simulink model "BLDC_motor"  (R2020b)
settings: Solver=VariableStepAuto  StartTime=0.0  StopTime=10.0  RelTol=1e-3
values from neighbouring files (symbols this model uses):
  f1 = 1    [costant_declaration.m]
  f2 = 2    [costant_declaration.m]
  f3 = 3    [costant_declaration.m]
  J = 0.005    [costant_declaration.m]
  ke = 0.5    [costant_declaration.m]
  kf = 1.38e-8    (= 1.38e-08)    [costant_declaration.m]
  L = 0.091e-3    (= 9.1e-05)    [costant_declaration.m]
  R = 12.50    (= 12.5)    [costant_declaration.m]
undefined symbols (not defined in the file or in its folder): Te, TL
settings Model: Creator=shraddha  LastModifiedBy=shraddha

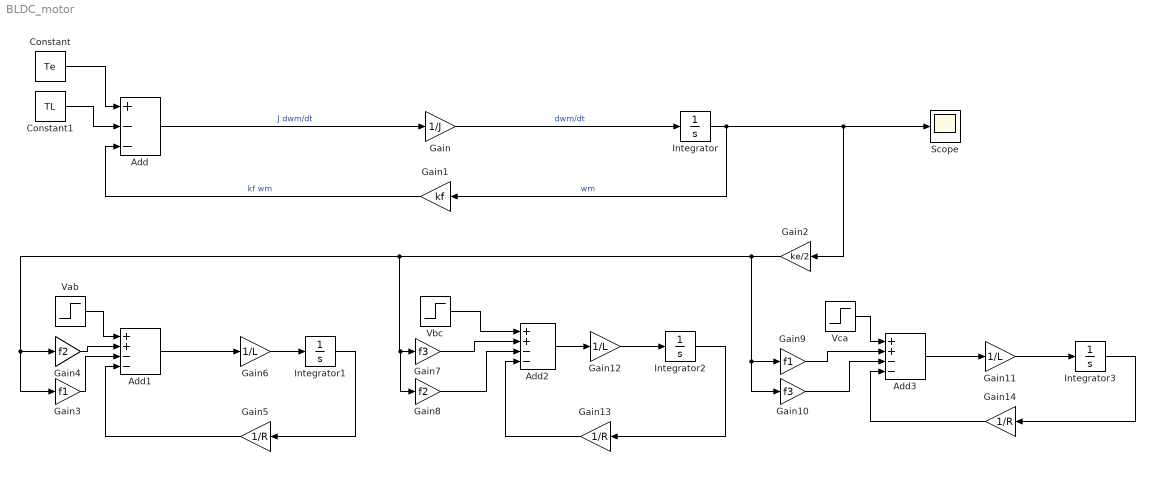
== system BLDC_motor ==
  Add : Sum  Inputs=+--
  Add1 : Sum  Inputs=++--
  Add2 : Sum  Inputs=++--
  Add3 : Sum  Inputs=++--
  Constant : Constant  Value=Te
  Constant1 : Constant  Value=TL
  Gain : Gain  Gain=1/J
  Gain1 : Gain  Gain=kf
  Gain10 : Gain  Gain=f3
  Gain11 : Gain  Gain=1/L
  Gain12 : Gain  Gain=1/L
  Gain13 : Gain  Gain=1/R
  Gain14 : Gain  Gain=1/R
  Gain2 : Gain  Gain=ke/2
  Gain3 : Gain  Gain=f1
  Gain4 : Gain  Gain=f2
  Gain5 : Gain  Gain=1/R
  Gain6 : Gain  Gain=1/L
  Gain7 : Gain  Gain=f3
  Gain8 : Gain  Gain=f2
  Gain9 : Gain  Gain=f1
  Integrator{,1..3} (4 alike) : Integrator
  Scope : Scope
  Vab : Step  SampleTime=0
  Vbc : Step  SampleTime=0
  Vca : Step  SampleTime=0
  wires:
  Add/1 -> Gain/1  "J dwm/dt"
  Gain/1 -> Integrator/1  "dwm/dt"
  Integrator/1 -> Gain2/1, Scope/1, Gain1/1  "wm"
  Gain1/1 -> Add/3  "kf wm"
  Constant1/1 -> Add/2
  Constant/1 -> Add/1
  Gain6/1 -> Integrator1/1
  Add1/1 -> Gain6/1
  Vab/1 -> Add1/1
  Integrator1/1 -> Gain5/1
  Gain5/1 -> Add1/4
  Gain2/1 -> Gain8/1, Gain7/1, Gain3/1, Gain4/1, Gain9/1, Gain10/1
  Gain3/1 -> Add1/3
  Gain4/1 -> Add1/2
  Vbc/1 -> Add2/1
  Add3/1 -> Gain11/1
  Gain11/1 -> Integrator3/1
  Vca/1 -> Add3/1
  Integrator3/1 -> Gain14/1
  Gain14/1 -> Add3/4
  Gain9/1 -> Add3/2
  Gain10/1 -> Add3/3
  Gain7/1 -> Add2/2
  Gain8/1 -> Add2/3
  Gain13/1 -> Add2/4
  Add2/1 -> Gain12/1
  Integrator2/1 -> Gain13/1
  Gain12/1 -> Integrator2/1
